simulink model "first_order_tuning"  (R2016b)
settings: Solver=FixedStepAuto  StartTime=0.0  StopTime=300  FixedStep=1  RelTol=1e-3
values from neighbouring files (symbols this model uses):
  bat_energy = bat_energy_kwh*1000*3600    (= 216000000)    [Init_PI_reg.m]    (also in Initial_test.m; battery_test_res.mat; body_test_res.mat; motor_test_res.mat)
  g = 9.80665    [Init_PI_reg.m]    (also in Initial_test.m; battery_test_res.mat; body_test_res.mat; motor_test_res.mat)
  inverter_eff = 0.93    [Init_PI_reg.m]    (also in Initial_test.m; battery_test_res.mat; body_test_res.mat; motor_test_res.mat)
  k_drag = (1/2)*air_density*SCx    (= 0.435741)    [Init_PI_reg.m]    (also in Initial_test.m; battery_test_res.mat; body_test_res.mat; motor_test_res.mat)
  k_rolling = 0.013*m*g    (= 224.376152)    [Init_PI_reg.m]    (also in Initial_test.m; battery_test_res.mat; body_test_res.mat; motor_test_res.mat)
  m = 1600+80*2    (= 1760)    [Init_PI_reg.m]    (also in Initial_test.m; battery_test_res.mat; body_test_res.mat; motor_test_res.mat)
  motor_eff = 0.91    [Init_PI_reg.m]    (also in Initial_test.m; battery_test_res.mat; body_test_res.mat; motor_test_res.mat)
  mps_to_kmph = 3.6    [Init_PI_reg.m]    (also in Initial_test.m; battery_test_res.mat; body_test_res.mat; motor_test_res.mat)
  power_max = 160e3    (= 160000)    [Init_PI_reg.m]    (also in Initial_test.m; battery_test_res.mat; body_test_res.mat; motor_test_res.mat)
  rmp_2_kmph = (kmph_max/rpm_max)    (= 0.0136892539357)    [Init_PI_reg.m]    (also in Initial_test.m; battery_test_res.mat; body_test_res.mat; motor_test_res.mat)
  soc = [0, 2, 6, 9, 20, 37, 42, 57, 66, 77, 85, 91, 95, 98, 100]    [Init_PI_reg.m]    (also in Initial_test.m; battery_test_res.mat = [0 2 6 9 20 37 42 57 66 77 85 91 ... (15 elements, 1x15)]; body_test_res.mat = [0 2 6 9 20 37 42 57 66 77 85 91 ... (15 elements, 1x15)]; motor_test_res.mat = [0 2 6 9 20 37 42 57 66 77 85 91 ... (15 elements, 1x15)])
  torque_max = 300    [Init_PI_reg.m]    (also in Initial_test.m; battery_test_res.mat; body_test_res.mat; motor_test_res.mat)
  tourque_2_thrust = (2*pi*3.6/60)/rmp_2_kmph    (= 27.5392012014)    [Init_PI_reg.m]    (also in Initial_test.m; battery_test_res.mat; body_test_res.mat; motor_test_res.mat)
  U_bat = U_cell*Nb_serial    [Init_PI_reg.m]    (also in Initial_test.m; battery_test_res.mat = [327.36 346.56 362.88 370.56 373.44 374.4 376.32 381.12 384 ; body_test_res.mat = [327.36 346.56 362.88 370.56 373.44 374.4 376.32 381.12 384 ; motor_test_res.mat = [327.36 346.56 362.88 370.56 373.44 374.4 376.32 381.12 384 )
  U_uvp = 330    [Init_PI_reg.m]    (also in Initial_test.m; battery_test_res.mat; body_test_res.mat; motor_test_res.mat)
  Velocity_0 = 0    [Init_PI_reg.m]    (also in Initial_test.m; battery_test_res.mat; body_test_res.mat; motor_test_res.mat)
settings Model: Creator=a037702  LastModifiedBy=a037702

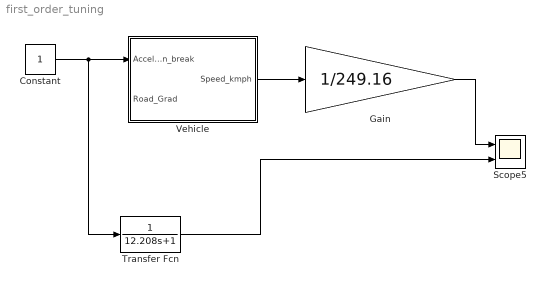
== system first_order_tuning ==
  Constant : Constant
  Gain : Gain  Gain=1/249.16
  Scope5 : Scope  NumInputPorts=2
  Transfer Fcn : TransferFcn  Denominator=[12.208 1]
  Vehicle : Subsystem
  wires:
  Vehicle/1(Speed_kmph) -> Gain/1
  Transfer Fcn/1 -> Scope5/2
  Constant/1 -> Transfer Fcn/1, Vehicle/1(Acceleration_break)
  Gain/1 -> Scope5/1

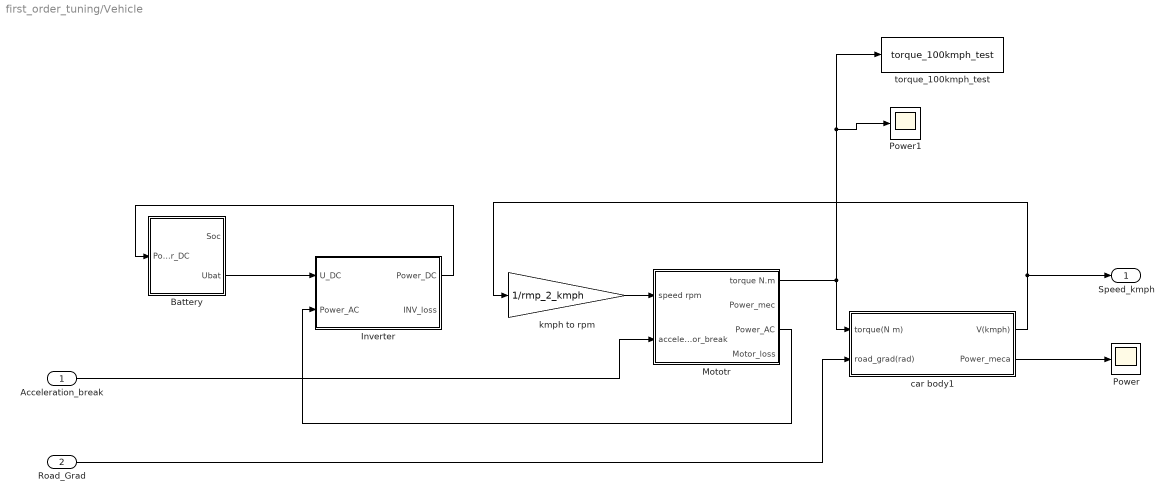
== system first_order_tuning/Vehicle ==
  Acceleration_break : Inport
  Road_Grad : Inport  Port=2
  Battery : Subsystem
  Inverter : Subsystem
  Mototr : Subsystem
  Power : Scope
  Power1 : Scope
  car body1 : Subsystem
  kmph to rpm : Gain  Gain=1/rmp_2_kmph
  torque_100kmph_test : ToWorkspace  VariableName=torque_100kmph_test  SaveFormat=Structure With Time  SampleTime=-1
      settings: Save2DSignal=2-D array (concatenate along first dimension)
  Speed_kmph : Outport
  wires:
  Battery/2(Ubat) -> Inverter/1(U_DC)
  Inverter/1(Power_DC) -> Battery/1(Power_DC)
  Acceleration_break/1 -> Mototr/2(accelerator_break)
  Road_Grad/1 -> car body1/2(road_grad(rad))
  Mototr/1(torque N.m) -> car body1/1(torque(N m)), Power1/1, torque_100kmph_test/1
  kmph to rpm/1 -> Mototr/1(speed rpm)
  car body1/1(V(kmph)) -> Speed_kmph/1, kmph to rpm/1
  car body1/2(Power_meca) -> Power/1
  Mototr/3(Power_AC) -> Inverter/2(Power_AC)

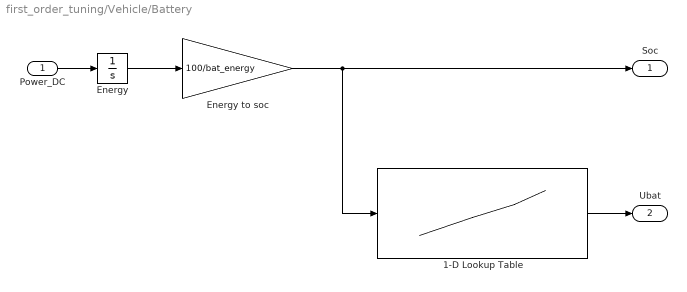
== system first_order_tuning/Vehicle/Battery ==
  Power_DC : Inport
  1-D Lookup Table : Lookup_n-D  NumberOfTableDimensions=1  BreakpointsForDimension1=soc  BreakpointsForDimension1DataTypeStr=double  Table=U_bat  TableDataTypeStr=double  InternalRulePriority=Speed  RndMeth=Simplest  InputSameDT=on
  Energy : Integrator  InitialCondition=bat_energy  LimitOutput=on  UpperSaturationLimit=bat_energy  LowerSaturationLimit=0
  Energy to soc : Gain  Gain=100/bat_energy
  Soc : Outport
  Ubat : Outport  Port=2
  wires:
  Energy/1 -> Energy to soc/1
  Energy to soc/1 -> 1-D Lookup Table/1, Soc/1
  Power_DC/1 -> Energy/1
  1-D Lookup Table/1 -> Ubat/1

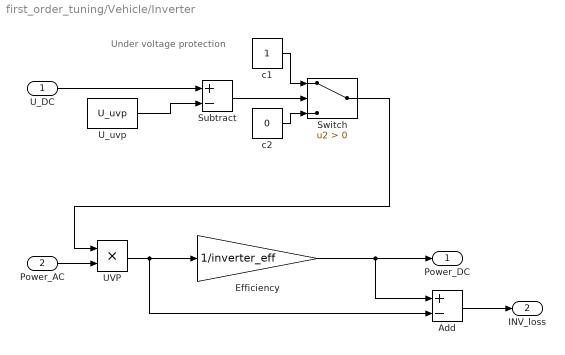
== system first_order_tuning/Vehicle/Inverter ==
  note: Under voltage protection
  U_DC : Inport
  Power_AC : Inport  Port=2
  Add : Sum  Inputs=+-
  Efficiency : Gain  Gain=1/inverter_eff
  Subtract : Sum  Inputs=+-
  Switch : Switch  Criteria=u2 > Threshold
  UVP : Product
  U_uvp : Constant  Value=U_uvp
  c1 : Constant
  c2 : Constant  Value=0
  Power_DC : Outport
  INV_loss : Outport  Port=2
  wires:
  UVP/1 -> Efficiency/1, Add/2
  Add/1 -> INV_loss/1
  U_uvp/1 -> Subtract/2
  U_DC/1 -> Subtract/1
  Subtract/1 -> Switch/2
  Efficiency/1 -> Power_DC/1, Add/1
  Switch/1 -> UVP/1
  c1/1 -> Switch/1
  c2/1 -> Switch/3
  Power_AC/1 -> UVP/2

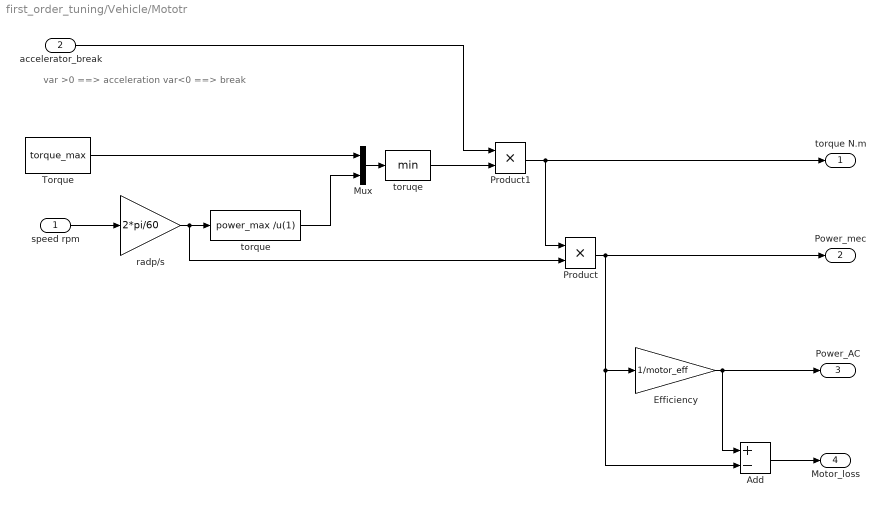
== system first_order_tuning/Vehicle/Mototr ==
  note: var >0 ==> acceleration var<0 ==> break
  speed rpm : Inport
  accelerator_break : Inport  Port=2
  Add : Sum  Inputs=+-
  Efficiency : Gain  Gain=1/motor_eff
  Mux : Mux  Inputs=2
  Product : Product
  Product1 : Product
  Torque : Constant  Value=torque_max
  radp/s : Gain  Gain=2*pi/60
  torque : Fcn  Expr=power_max /u(1)
  toruqe : MinMax
  torque N.m : Outport
  Power_mec : Outport  Port=2
  Power_AC : Outport  Port=3
  Motor_loss : Outport  Port=4
  wires:
  Product1/1 -> Product/1, torque N.m/1
  Mux/1 -> toruqe/1
  Torque/1 -> Mux/1
  radp/s/1 -> Product/2, torque/1
  torque/1 -> Mux/2
  speed rpm/1 -> radp/s/1
  Product/1 -> Add/2, Efficiency/1, Power_mec/1
  Efficiency/1 -> Add/1, Power_AC/1
  Add/1 -> Motor_loss/1
  toruqe/1 -> Product1/2
  accelerator_break/1 -> Product1/1

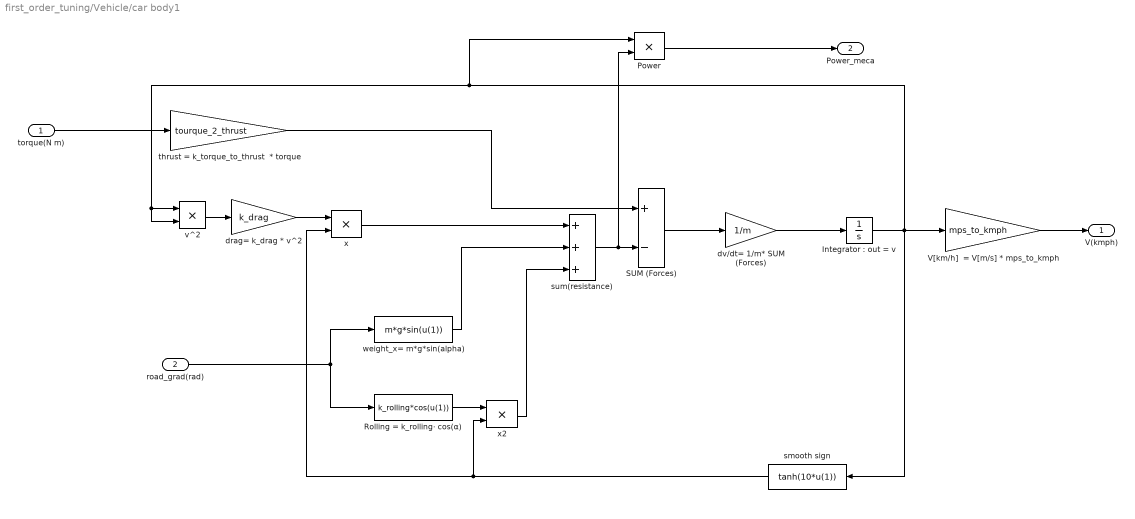
== system first_order_tuning/Vehicle/car body1 ==
  torque(N m) : Inport
  road_grad(rad) : Inport  Port=2
  "Integrator : out = v" : Integrator  InitialCondition=Velocity_0  LimitOutput=on  UpperSaturationLimit=400  LowerSaturationLimit=-400
  Power : Product
  Rolling = k_rolling· cos(α) : Fcn  Expr=k_rolling*cos(u(1))
  SUM (Forces) : Sum  Inputs=+-
  V[km/h]  = V[m/s] * mps_to_kmph : Gain  Gain=mps_to_kmph
  drag= k_drag * v^2 : Gain  Gain=k_drag
  dv/dt= 1/m* SUM (Forces) : Gain  Gain=1/m
  smooth sign : Fcn  Expr=tanh(10*u(1))
  sum(resistance) : Sum  Inputs=+++
  thrust = k_torque_to_thrust  * torque : Gain  Gain=tourque_2_thrust
  v^2 : Product
  weight_x= m*g*sin(alpha) : Fcn  Expr=m*g*sin(u(1))
  "x " : Product
  x2 : Product
  V(kmph) : Outport
  Power_meca : Outport  Port=2
  wires:
  weight_x= m*g*sin(alpha)/1 -> sum(resistance)/2
  thrust = k_torque_to_thrust  * torque/1 -> SUM (Forces)/1
  v^2/1 -> drag= k_drag * v^2/1
  V[km/h]  = V[m/s] * mps_to_kmph/1 -> V(kmph)/1
  "Integrator : out = v"/1 -> smooth sign/1, V[km/h]  = V[m/s] * mps_to_kmph/1, Power/1, v^2/2, v^2/1
  dv/dt= 1/m* SUM (Forces)/1 -> "Integrator : out = v"/1
  SUM (Forces)/1 -> dv/dt= 1/m* SUM (Forces)/1
  torque(N m)/1 -> thrust = k_torque_to_thrust  * torque/1
  "x "/1 -> sum(resistance)/1
  road_grad(rad)/1 -> Rolling = k_rolling· cos(α)/1, weight_x= m*g*sin(alpha)/1
  Power/1 -> Power_meca/1
  Rolling = k_rolling· cos(α)/1 -> x2/1
  x2/1 -> sum(resistance)/3
  drag= k_drag * v^2/1 -> "x "/1
  smooth sign/1 -> "x "/2, x2/2
  sum(resistance)/1 -> Power/2, SUM (Forces)/2
